simulink library "lib4"  (Simulink 6.0)
libraries: lib2 x1
settings Model: Creator=awarlock  LastModifiedBy=mshakeri  ExtModeAutoUpdateStatusClock=off

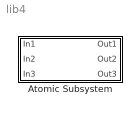
== system lib4 ==
  Atomic Subsystem : Subsystem  TreatAsAtomicUnit=on

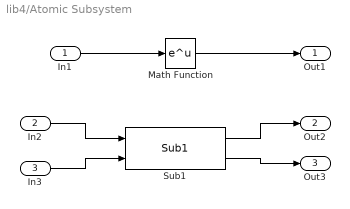
== system lib4/Atomic Subsystem ==
  In1 : Inport
  In2 : Inport  Port=2
  In3 : Inport  Port=3
  Math Function : Math  SaturateOnIntegerOverflow=on
  Sub1 : lib2/Sub1  TreatAsAtomicUnit=on  SimViewingDevice=off  DataTypeOverride=UseLocalSettings  MinMaxOverflowLogging=UseLocalSettings
      settings: Permissions=ReadWrite  RTWFcnNameOpts=Auto  RTWFileNameOpts=Auto
  Out1 : Outport
  Out2 : Outport  Port=2
  Out3 : Outport  Port=3
  wires:
  In1/1 -> Math Function/1
  In2/1 -> Sub1/1
  In3/1 -> Sub1/2
  Sub1/1 -> Out2/1
  Sub1/2 -> Out3/1
  Math Function/1 -> Out1/1
